simulink model "simulinkur10"  (R2020a)
settings: Solver=ode1  StartTime=0.0  StopTime=7  FixedStep=0.001  RelTol=1e-3
values from neighbouring files (symbols this model uses):
  qi = [pi/2,0,pi/2,0,pi/2,pi/6]    [UR10code.m]
settings Model: Creator=zahra  LastModifiedBy=zahra
settings DataIOCC: ReturnWorkspaceOutputs=off

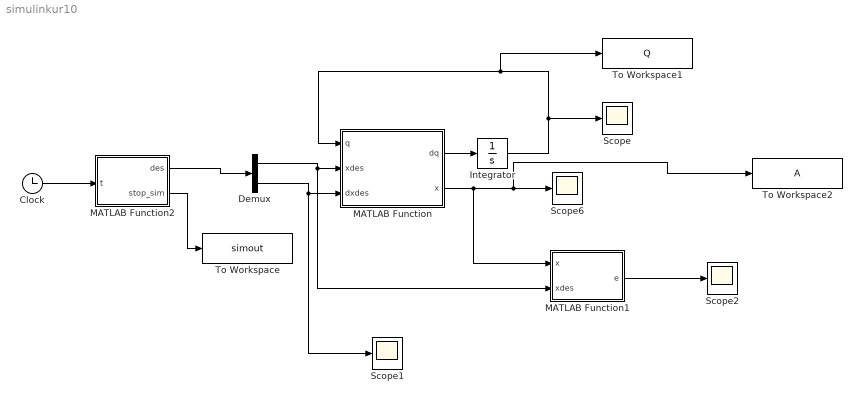
== system simulinkur10 ==
  Clock : Clock
  Demux : Demux  Outputs=2
  Integrator : Integrator  InitialCondition=qi
  MATLAB Function : MATLAB Function  TreatAsAtomicUnit=on
  MATLAB Function1 : MATLAB Function  TreatAsAtomicUnit=on
  MATLAB Function2 : MATLAB Function  TreatAsAtomicUnit=on
  Scope{,1..2,6} (4 alike) : Scope
  To Workspace : ToWorkspace  VariableName=simout  SaveFormat=Timeseries  SampleTime=-1
  To Workspace1 : ToWorkspace  VariableName=Q  SampleTime=-1
  To Workspace2 : ToWorkspace  VariableName=A  SampleTime=-1
  wires:
  Clock/1 -> MATLAB Function2/1(t)
  Demux/1 -> MATLAB Function1/2(xdes), MATLAB Function/2(xdes)
  Demux/2 -> Scope1/1, MATLAB Function/3(dxdes)
  MATLAB Function/1(dq) -> Integrator/1
  Integrator/1 -> Scope/1, To Workspace1/1, MATLAB Function/1(q)
  MATLAB Function2/1(des) -> Demux/1
  MATLAB Function2/2(stop_sim) -> To Workspace/1
  MATLAB Function/2(x) -> MATLAB Function1/1(x), To Workspace2/1, Scope6/1
  MATLAB Function1/1(e) -> Scope2/1

== matlab function simulinkur10/MATLAB Function1 ==
  data: x input; e output; xdes input
function e = eroe(x,xdes)

e=xdes-x;

== matlab function simulinkur10/MATLAB Function ==
  data: q input; xdes input; dq output; dxdes input; x output
 
function [dq,x]=control(q,xdes,dxdes)
q1=q(1);q2=q(2);q3=q(3);q4=q(4);q5=q(5);q6=q(6);
 
E=[- cos(q6)*(sin(q1)*sin(q5) - cos(q5)*(cos(q4)*(cos(q1)*cos(q2)*cos(q3) - cos(q1)*sin(q2)*sin(q3)) - sin(q4)*(cos(q1)*cos(q2)*sin(q3) + cos(q1)*cos(q3)*sin(q2)))) - sin(q6)*(cos(q4)*(cos(q1)*cos(q2)*sin(q3) + cos(q1)*cos(q3)*sin(q2)) + sin(q4)*(cos(q1)*cos(q2)*cos(q3) - cos(q1)*sin(q2)*sin(q3))),   sin(q6)*(sin(q1)*sin(q5) - cos(q5)*(cos(q4)*(cos(q1)*cos(q2)*cos(q3) - cos(q1)*sin(q2)*sin(q3)) - sin(q4)*(cos(q1)*cos(q2)*sin(q3) + cos(q1)*cos(q3)*sin(q2)))) - cos(q6)*(cos(q4)*(cos(q1)*cos(q2)*sin(q3) + cos(q1)*cos(q3)*sin(q2)) + sin(q4)*(cos(q1)*cos(q2)*cos(q3) - cos(q1)*sin(q2)*sin(q3))), - cos(q5)*sin(q1) - sin(q5)*(cos(q4)*(cos(q1)*cos(q2)*cos(q3) - cos(q1)*sin(q2)*sin(q3)) - sin(q4)*(cos(q1)*cos(q2)*sin(q3) + cos(q1)*cos(q3)*sin(q2)))
   cos(q6)*(cos(q1)*sin(q5) - cos(q5)*(cos(q4)*(sin(q1)*sin(q2)*sin(q3) - cos(q2)*cos(q3)*sin(q1)) + sin(q4)*(cos(q2)*sin(q1)*sin(q3) + cos(q3)*sin(q1)*sin(q2)))) - sin(q6)*(cos(q4)*(cos(q2)*sin(q1)*sin(q3) + cos(q3)*sin(q1)*sin(q2)) - sin(q4)*(sin(q1)*sin(q2)*sin(q3) - cos(q2)*cos(q3)*sin(q1))), - sin(q6)*(cos(q1)*sin(q5) - cos(q5)*(cos(q4)*(sin(q1)*sin(q2)*sin(q3) - cos(q2)*cos(q3)*sin(q1)) + sin(q4)*(cos(q2)*sin(q1)*sin(q3) + cos(q3)*sin(q1)*sin(q2)))) - cos(q6)*(cos(q4)*(cos(q2)*sin(q1)*sin(q3) + cos(q3)*sin(q1)*sin(q2)) - sin(q4)*(sin(q1)*sin(q2)*sin(q3) - cos(q2)*cos(q3)*sin(q1))),   cos(q1)*cos(q5) + sin(q5)*(cos(q4)*(sin(q1)*sin(q2)*sin(q3) - cos(q2)*cos(q3)*sin(q1)) + sin(q4)*(cos(q2)*sin(q1)*sin(q3) + cos(q3)*sin(q1)*sin(q2)))
                                                                                     - sin(q6)*(cos(q4)*(cos(q2)*cos(q3) - sin(q2)*sin(q3)) - sin(q4)*(cos(q2)*sin(q3) + cos(q3)*sin(q2))) - cos(q5)*cos(q6)*(cos(q4)*(cos(q2)*sin(q3) + cos(q3)*sin(q2)) + sin(q4)*(cos(q2)*cos(q3) - sin(q2)*sin(q3))),                                                                                       cos(q5)*sin(q6)*(cos(q4)*(cos(q2)*sin(q3) + cos(q3)*sin(q2)) + sin(q4)*(cos(q2)*cos(q3) - sin(q2)*sin(q3))) - cos(q6)*(cos(q4)*(cos(q2)*cos(q3) - sin(q2)*sin(q3)) - sin(q4)*(cos(q2)*sin(q3) + cos(q3)*sin(q2))),                                                     sin(q5)*(cos(q4)*(cos(q2)*sin(q3) + cos(q3)*sin(q2)) + sin(q4)*(cos(q2)*cos(q3) - sin(q2)*sin(q3)))];
 
 
e=rotm2eul(E,'xyz');

x =[ (1157*cos(q4)*(cos(q1)*cos(q2)*sin(q3) + cos(q1)*cos(q3)*sin(q2)))/10000 - (153*cos(q1)*cos(q2))/250 - (461*cos(q5)*sin(q1))/5000 - (1476649253021493*sin(q1))/9007199254740992 + (1157*sin(q4)*(cos(q1)*cos(q2)*cos(q3) - cos(q1)*sin(q2)*sin(q3)))/10000 - (461*sin(q5)*(cos(q4)*(cos(q1)*cos(q2)*cos(q3) - cos(q1)*sin(q2)*sin(q3)) - sin(q4)*(cos(q1)*cos(q2)*sin(q3) + cos(q1)*cos(q3)*sin(q2))))/5000 - (5723*cos(q1)*cos(q2)*cos(q3))/10000 + (5723*cos(q1)*sin(q2)*sin(q3))/10000
 (1476649253021493*cos(q1))/9007199254740992 + (461*cos(q1)*cos(q5))/5000 - (153*cos(q2)*sin(q1))/250 + (1157*cos(q4)*(cos(q2)*sin(q1)*sin(q3) + cos(q3)*sin(q1)*sin(q2)))/10000 - (1157*sin(q4)*(sin(q1)*sin(q2)*sin(q3) - cos(q2)*cos(q3)*sin(q1)))/10000 + (461*sin(q5)*(cos(q4)*(sin(q1)*sin(q2)*sin(q3) - cos(q2)*cos(q3)*sin(q1)) + sin(q4)*(cos(q2)*sin(q1)*sin(q3) + cos(q3)*sin(q1)*sin(q2))))/5000 + (5723*sin(q1)*sin(q2)*sin(q3))/10000 - (5723*cos(q2)*cos(q3)*sin(q1))/10000
                                                                                                                                                       (153*sin(q2))/250 + (5723*cos(q2)*sin(q3))/10000 + (5723*cos(q3)*sin(q2))/10000 + (461*sin(q5)*(cos(q4)*(cos(q2)*sin(q3) + cos(q3)*sin(q2)) + sin(q4)*(cos(q2)*cos(q3) - sin(q2)*sin(q3))))/5000 + (1157*cos(q4)*(cos(q2)*cos(q3) - sin(q2)*sin(q3)))/10000 - (1157*sin(q4)*(cos(q2)*sin(q3) + cos(q3)*sin(q2)))/10000 + 1273/10000
                                                                                                                                                       e(1)
                                                                                                                                                       e(2)
                                                                                                                                                       e(3)];
 
Jg =[ 0.612*cos(q2)*sin(q1) - 0.0922*cos(q1)*cos(q5) - 0.164*cos(q1) - 0.572*sin(q1)*sin(q2)*sin(q3) + 0.0922*cos(q2 + q3 + q4)*sin(q1)*sin(q5) - 0.116*cos(q2 + q3)*sin(q1)*sin(q4) - 0.116*sin(q2 + q3)*cos(q4)*sin(q1) + 0.572*cos(q2)*cos(q3)*sin(q1), cos(q1)*(0.572*sin(q2 + q3) + 0.612*sin(q2) + sin(q5)*(0.0922*cos(q2 + q3)*sin(q4) + 0.0922*sin(q2 + q3)*cos(q4)) + 0.116*cos(q2 + q3)*cos(q4) - 0.116*sin(q2 + q3)*sin(q4)),                        cos(q1)*(0.116*cos(q2 + q3 + q4) + 0.572*sin(q2 + q3) + 0.0922*sin(q2 + q3 + q4)*sin(q5)),                        cos(q1)*(0.116*cos(q2 + q3 + q4) + 0.0922*sin(q2 + q3 + q4)*sin(q5)),                        cos(q1)*(0.116*cos(q2 + q3 + q4) + 0.0922*sin(q2 + q3 + q4)*sin(q5)),                          0.0922*sin(q2 + q3 + q4)*cos(q1)*sin(q5)
 0.116*cos(q2 + q3)*cos(q1)*sin(q4) - 0.612*cos(q1)*cos(q2) - 0.0922*cos(q5)*sin(q1) - 0.0922*cos(q2 + q3 + q4)*cos(q1)*sin(q5) - 0.164*sin(q1) + 0.116*sin(q2 + q3)*cos(q1)*cos(q4) - 0.572*cos(q1)*cos(q2)*cos(q3) + 0.572*cos(q1)*sin(q2)*sin(q3), sin(q1)*(0.572*sin(q2 + q3) + 0.612*sin(q2) + sin(q5)*(0.0922*cos(q2 + q3)*sin(q4) + 0.0922*sin(q2 + q3)*cos(q4)) + 0.116*cos(q2 + q3)*cos(q4) - 0.116*sin(q2 + q3)*sin(q4)),                        sin(q1)*(0.116*cos(q2 + q3 + q4) + 0.572*sin(q2 + q3) + 0.0922*sin(q2 + q3 + q4)*sin(q5)),                        sin(q1)*(0.116*cos(q2 + q3 + q4) + 0.0922*sin(q2 + q3 + q4)*sin(q5)),                        sin(q1)*(0.116*cos(q2 + q3 + q4) + 0.0922*sin(q2 + q3 + q4)*sin(q5)),                          0.0922*sin(q2 + q3 + q4)*sin(q1)*sin(q5)
                                                                                                                                                                                                                                                   0,                                             0.0461*sin(q2 + q3 + q4 + q5) - 0.0461*sin(q2 + q3 + q4 - 1.0*q5) - 0.116*sin(q2 + q3 + q4) + 0.572*cos(q2 + q3) + 0.612*cos(q2), 0.0461*sin(q2 + q3 + q4 + q5) - 0.0461*sin(q2 + q3 + q4 - 1.0*q5) - 0.116*sin(q2 + q3 + q4) + 0.572*cos(q2 + q3), 0.0461*sin(q2 + q3 + q4 + q5) - 0.0461*sin(q2 + q3 + q4 - 1.0*q5) - 0.116*sin(q2 + q3 + q4), 0.0461*sin(q2 + q3 + q4 + q5) - 0.0461*sin(q2 + q3 + q4 - 1.0*q5) - 0.116*sin(q2 + q3 + q4), 0.0461*sin(q2 + q3 + q4 + q5) - 0.0461*sin(q2 + q3 + q4 - 1.0*q5)
                                                                                                                                                                                                                                                   0,                                                                                                                                                                 -1.0*sin(q1),                                                                                                     -1.0*sin(q1),                                                                                -1.0*sin(q1),                                                                   sin(q2 + q3 + q4)*cos(q1),     - 1.0*cos(q5)*sin(q1) - 1.0*cos(q2 + q3 + q4)*cos(q1)*sin(q5)
                                                                                                                                                                                                                                                   0,                                                                                                                                                                      cos(q1),                                                                                                          cos(q1),                                                                                     cos(q1),                                                                   sin(q2 + q3 + q4)*sin(q1),           cos(q1)*cos(q5) - 1.0*cos(q2 + q3 + q4)*sin(q1)*sin(q5)
                                                                                                                                                                                                                                                 1.0,                                                                                                                                                                            0,                                                                                                                0,                                                                                           0,                                                                           cos(q2 + q3 + q4),                                         sin(q2 + q3 + q4)*sin(q5)];
 
I=eye(3);
o=zeros(3);
T=[1 0 sin(e(2)) ;0  cos(e(1))  -cos(e(2))*sin(e(1)) ;0 sin(e(1)) cos(e(2))*cos(e(1))];
U=[I,o;o,T];

J=inv(U)*Jg;

 d=abs(det(J));
if d >= 0.4
    landa=0;
else
    landa=(1-(d/0.2)^2)*0.1;
end

dq=J'*inv(J*J'+landa*eye(6))*(dxdes+2000*eye(6)*(xdes-x));

end

== matlab function simulinkur10/MATLAB Function2 ==
  data: t input; des output; stop_sim output
function [des,stop_sim]=desire(t)
stop_sim=0;
xi=[-0.1639 ;-0.4963; 0.7918;0     ;    0  ; -2.6180];
xf=[-0.4645;-0.2327;0.3664;0    ;     0  ; -2.6180];

L=norm(xi-xf);
T=7;
vmax=0.1;
Ts=T-(L/vmax);
amax=vmax/Ts;
if t >= 0 && t <= Ts
    sig=amax*t^2/2;
    dsig=amax*t;
elseif t >= Ts && t <= (T-Ts)
    sig=vmax*t-vmax^2/(2*amax);
    dsig=vmax;
elseif t >=(T-Ts) && t <= T
    sig=-amax*(t-T)^2/2+vmax*T-vmax^2/amax;
    dsig=-amax*(t-T);
else
    sig=L;
    dsig=0;
    stop_sim=1;
end
xdes=xi+sig/L.*(xf-xi);
dxdes=dsig/L.*(xf-xi);
des=[xdes;dxdes];
